simulink model "galton_gen_sf"  (Simulink 8.1)
settings: Solver=FixedStepDiscrete  StartTime=0.0  StopTime=10.0  FixedStep=0.1  RelTol=1e-3
settings Model: Creator=zhan  LastModifiedBy=zhihan
settings DebuggingCC: StrictBusMsg=Warning
settings SFSimCC: SimParseCustomCode=off

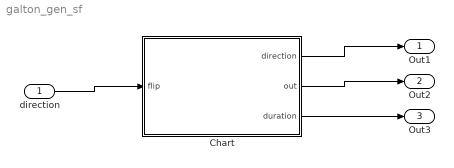
== system galton_gen_sf ==
  direction : Inport
  Chart : Stateflow chart  TreatAsAtomicUnit=on
  Out1 : Outport
  Out2 : Outport  Port=2
  Out3 : Outport  Port=3
  wires:
  direction/1 -> Chart/1(flip)
  Chart/1(direction) -> Out1/1
  Chart/2(out) -> Out2/1
  Chart/3(duration) -> Out3/1

== stateflow chart Chart ==
  settings: updateMethod=DISCRETE  sampleTime=0.1
  state falling
    entry:
    duration=1;
    out = 2;
  (default) -> falling : /direction=0;
  (junction 8) -> falling [order 1] : [flip==1]/direction=1;
  (junction 8) -> falling [order 2] : [flip==2]/direction=-1;
  falling -> (junction 8) : after(duration*10, tick)
  data: flip input double; direction output double; out output double; duration output double
